simulink model "controlador"  (R2025a)
settings: Solver=VariableStepAuto  StartTime=0.0  StopTime=10.0  RelTol=1e-3
settings Model: Creator=skynet  LastModifiedBy=skynet

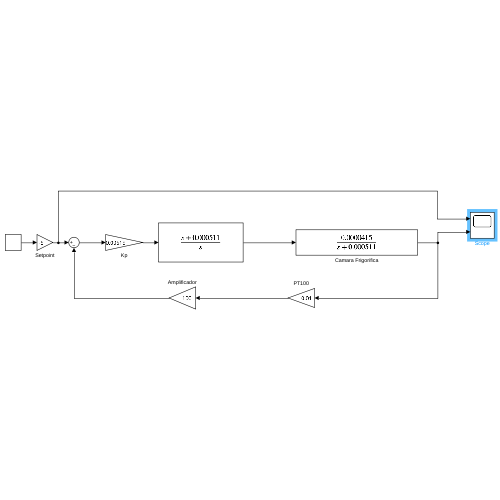
[thumbnail: Simulink's stored preview of the top-level diagram]
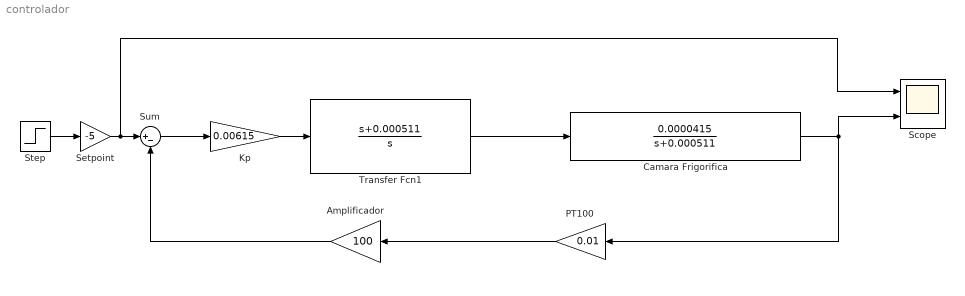
== system controlador ==
  Amplificador : Gain  Gain=100
  Camara Frigorifica : TransferFcn  Numerator=[0.0000415]  Denominator=[1, 0.000511]
  Kp : Gain  Gain=0.00615
  PT100 : Gain  Gain=0.01
  Scope : Scope  NumInputPorts=2
      settings: ActiveDisplayYMinimum=-222.20045450728077  ActiveDisplayYMaximum=177.73746177814104
  Setpoint : Gain  Gain=-5
  Step : Step  After=30  SampleTime=0
  Sum : Sum  Inputs=|+-
  Transfer Fcn1 : TransferFcn  Numerator=[1 0.000511]  Denominator=[1 0 ]
  wires:
  Amplificador/1 -> Sum/2
  PT100/1 -> Amplificador/1
  Step/1 -> Setpoint/1
  Sum/1 -> Kp/1
  Kp/1 -> Transfer Fcn1/1
  Transfer Fcn1/1 -> Camara Frigorifica/1
  Setpoint/1 -> Sum/1, Scope/1
  Camara Frigorifica/1 -> Scope/2, PT100/1
